simulink model "plat_ts"  (R2018b)
settings: Solver=VariableStepAuto  StartTime=0.0  StopTime=10.0  RelTol=1e-3
undefined symbols (not defined in the file or in its folder): plat
undefined symbols (not defined in the file): teth1, teth2, teth3
libraries: forceTether x3, forceGravBuoy x2, actuatorForces x1
settings Model: Creator=embeato2  LastModifiedBy=embeato2

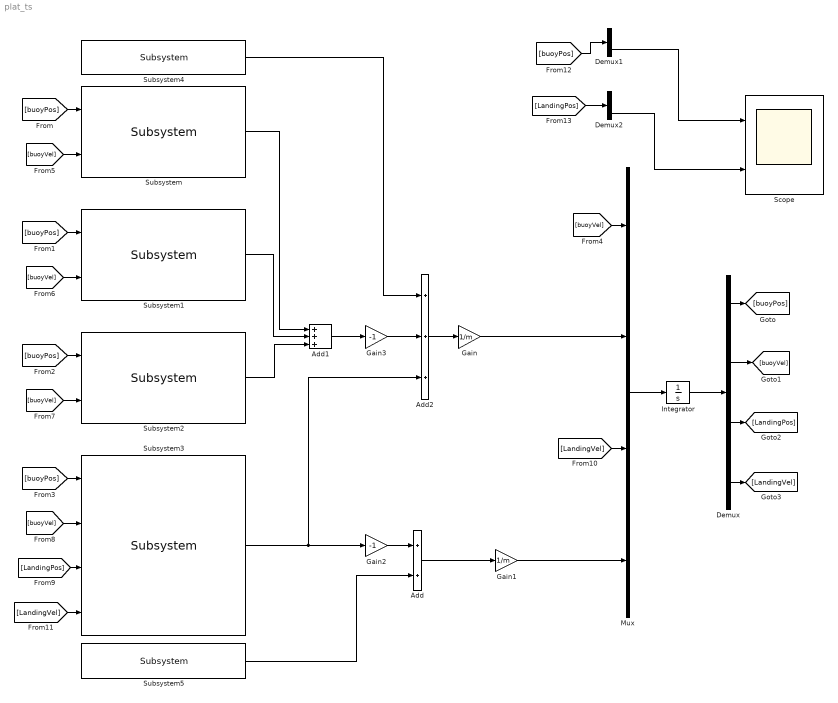
== system plat_ts ==
  Add : Sum
  Add1 : Sum  Inputs=+++
  Add2 : Sum  Inputs=+++
  Demux : Demux
  Demux1 : Demux  Outputs=3
  Demux2 : Demux  Outputs=3
  Gain : Gain  Gain=1/m  mask{m=plat.buoy.mass.Value}
      mask prompts: m "Mass of Buoyant Platform"
  Gain1 : Gain  Gain=1/m  mask{m=plat.landing.mass.Value}
      mask prompts: m "Mass of Buoyant Platform"
  Gain2 : Gain  Gain=-1
  Gain3 : Gain  Gain=-1
  Integrator : Integrator  InitialCondition=plat.initial.Value
  Mux : Mux
  Scope : Scope  NumInputPorts=2
  Subsystem : forceTether/Subsystem  mask{cmDistance=teth1.cmDistanceBuoy, anchorPosition=teth1.anchorPos, unstretched=teth1.unstretchedL, k=teth1.k, b=teth1.b}
      mask prompts: cmDistance "Distance of Center of Mass"; anchorPosition "Anchor Position"; unstretched "Unstretched Length"
  Subsystem1 : forceTether/Subsystem  mask{cmDistance=teth2.cmDistanceBuoy, anchorPosition=teth2.anchorPos, unstretched=teth2.unstretchedL, k=teth2.k, b=teth2.b}
      mask prompts: cmDistance "Distance of Center of Mass"; anchorPosition "Anchor Position"; unstretched "Unstretched Length"
  Subsystem2 : forceTether/Subsystem  mask{cmDistance=teth3.cmDistanceBuoy, anchorPosition=teth3.anchorPos, unstretched=teth3.unstretchedL, k=teth3.k, b=teth3.b}
      mask prompts: cmDistance "Distance of Center of Mass"; anchorPosition "Anchor Position"; unstretched "Unstretched Length"
  Subsystem3 : actuatorForces/Subsystem  mask{k=plat.actuator.k.Value, b=plat.actuator.b.Value, unstretchedL=plat.actuator.unstretchedL.Value}
      mask prompts: k "Spring Constant of Acutator"; b "Damping Constant"; unstretchedL "Unstretched Length"
  Subsystem4 : forceGravBuoy/Subsystem  mask{g=plat.env.g.Value, mass=plat.buoy.mass.Value, rho=plat.env.rho.Value, volume=plat.buoy.vol.Value}
      mask prompts: g "Gravity"; rho "Density of Fluid (Air = 0)"
  Subsystem5 : forceGravBuoy/Subsystem  mask{g=plat.env.g.Value, mass=plat.landing.mass.Value, rho=0, volume=plat.landing.vol.Value}
      mask prompts: g "Gravity"; rho "Density of Fluid (Air = 0)"
  wires:
  Gain/1 -> Mux/2
  Gain1/1 -> Mux/4
  Mux/1 -> Integrator/1
  Subsystem/1 -> Add1/1
  Subsystem1/1 -> Add1/2
  Subsystem2/1 -> Add1/3
  Subsystem3/1 -> Add2/3, Gain2/1
  Add/1 -> Gain1/1
  Subsystem5/1 -> Add/2
  Gain2/1 -> Add/1
  Add2/1 -> Gain/1
  Add1/1 -> Gain3/1
  Subsystem4/1 -> Add2/1
  Integrator/1 -> Demux/1
  Demux/1 -> [buoyPos]
  [buoyPos] -> Subsystem/1
  [buoyPos] -> Subsystem1/1
  [buoyPos] -> Subsystem2/1
  [buoyPos] -> Subsystem3/1
  Demux/2 -> [buoyVel]
  [buoyVel] -> Mux/1
  [buoyVel] -> Subsystem/2
  [buoyVel] -> Subsystem1/2
  [buoyVel] -> Subsystem2/2
  [buoyVel] -> Subsystem3/2
  Demux/3 -> [LandingPos]
  [LandingPos] -> Subsystem3/3
  Demux/4 -> [LandingVel]
  [LandingVel] -> Mux/3
  [LandingVel] -> Subsystem3/4
  [buoyPos] -> Demux1/1
  Demux1/3 -> Scope/1
  [LandingPos] -> Demux2/1
  Demux2/3 -> Scope/2
  Gain3/1 -> Add2/2
